simulink model "Closed_Loop_With_PID_Neural_for_Attitude_plant_predcont"  (R2018b)
settings: Solver=ode45  StartTime=0.0  StopTime=100  FixedStep=0.0001  RelTol=1e3  SampleTimeConstraint=STIndependent  EnableMultiTasking=on
undefined symbols (not defined in the file): DiscIntNeverNeededParam
libraries: dspmtrx3 x6, neural x3, vrlib x2, sharedutil x1, slrtlib x1
CloseFcn:
  | rtwprivate ssgencode ModelCloseRequest controller
settings Model: Creator=acer  LastModifiedBy=the other guy
settings SolverCC: ZeroCrossControl=DisableAll  AutoInsertRateTranBlk=on
settings DataIOCC: LimitDataPoints=on  SaveFormat=Array  SignalLoggingSaveFormat=ModelDataLogs
settings OptimizationCC: ExpressionDepthLimit=2147483647  LifeSpan=inf
settings DebuggingCC: SaveWithParameterizedLinksMsg=none  UnderspecifiedInitializationDetection=Classic  MergeDetectMultiDrivingBlocksExec=none  SolverPrmCheckMsg=warning  FcnCallInpInsideContextMsg=warning  StateNameClashWarn=warning  SFUnexpectedBacktrackingDiag=warning  SFNoUnconditionalDefaultTransitionDiag=warning  SFExecutionAtInitializationDiag=none
settings HardwareCC: ProdBitPerPointer=32  ProdBitPerSizeT=32  ProdBitPerPtrDiffT=32  ProdLargestAtomicFloat=None  ProdIntDivRoundTo=Undefined  ProdEndianess=Unspecified  ProdWordSize=32  ProdHWDeviceType=32-bit Generic
settings ModelReferenceCC: PropagateSignalLabelsOutOfModel=off
settings SFSimCC: SimUseLocalCustomCode=off
settings RTWCC: RTWUseLocalCustomCode=off
settings CodeAppCC: StateflowObjectComments=on
settings GRTTargetCC: TargetLangStandard=C89/C90 (ANSI)  GeneratePreprocessorConditionals=Disable all  CombineOutputUpdateFcns=off  GRTInterface=on
settings ConfigComp: CovMetricSettings=dw  CovHtmlReporting=on  CovSaveCumulativeToWorkspaceVar=on  CovSaveSingleToWorkspaceVar=on  CovExternalEMLEnable=off

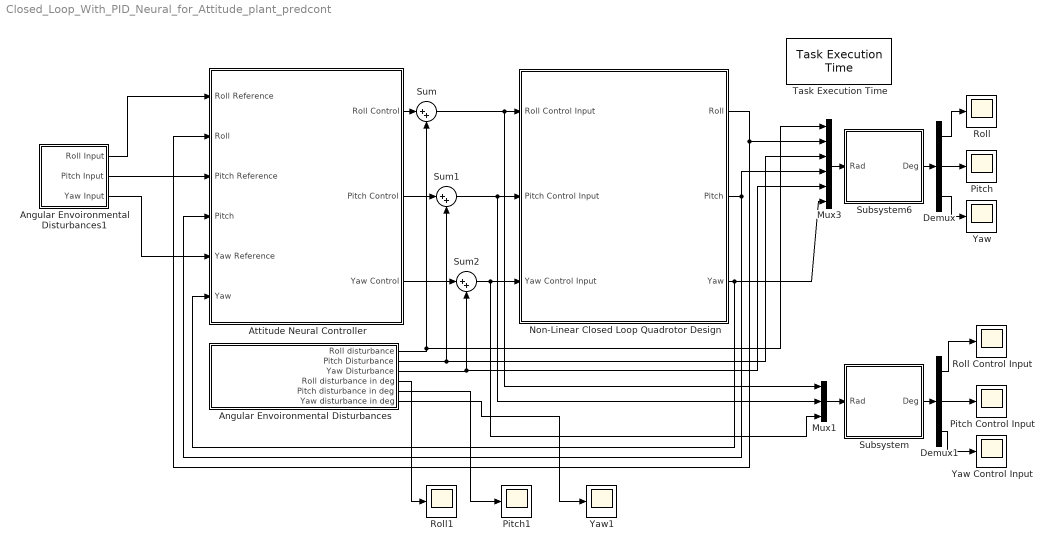
== system Closed_Loop_With_PID_Neural_for_Attitude_plant_predcont ==
  Angular Envoironmental Disturbances : Subsystem
  Angular Envoironmental Disturbances1 : Subsystem
  Attitude Neural Controller : Subsystem
  Demux : Demux  Outputs=[2,2,2]
  Demux1 : Demux  Outputs=3
  Mux1 : Mux  Inputs=3
  Mux3 : Mux  Inputs=6
  Non-Linear Closed Loop Quadrotor Design : Subsystem
  Pitch : Scope
  Pitch Control Input : Scope
  Pitch1 : Scope
  Roll : Scope
  Roll Control Input : Scope
  Roll1 : Scope
  Subsystem : Subsystem
  Subsystem6 : Subsystem
  Sum : Sum  Inputs=|++
  Sum1 : Sum  Inputs=|++
  Sum2 : Sum  Inputs=|++
  "Task Execution Time " : slrtlib/Target Management/Execution Parameters/Task Execution Time   ts=0.001
      settings: SourceProductName=Simulink Real-Time  SourceProductBaseCode=XP
  Yaw : Scope
  Yaw Control Input : Scope
  Yaw1 : Scope
  wires:
  Non-Linear Closed Loop Quadrotor Design/1(Roll) -> Mux3/2, Attitude Neural Controller/2(Roll)
  Angular Envoironmental Disturbances1/1(Roll Input) -> Attitude Neural Controller/1(Roll Reference)
  Demux1/1 -> Roll Control Input/1
  Angular Envoironmental Disturbances1/2(Pitch Input) -> Attitude Neural Controller/3(Pitch Reference)
  Non-Linear Closed Loop Quadrotor Design/2(Pitch) -> Attitude Neural Controller/4(Pitch), Mux3/4
  Demux1/2 -> Pitch Control Input/1
  Sum1/1 -> Mux1/2, Non-Linear Closed Loop Quadrotor Design/2(Pitch Control Input)
  Sum/1 -> Mux1/1, Non-Linear Closed Loop Quadrotor Design/1(Roll Control Input)
  Sum2/1 -> Mux1/3, Non-Linear Closed Loop Quadrotor Design/3(Yaw Control Input)
  Non-Linear Closed Loop Quadrotor Design/3(Yaw) -> Attitude Neural Controller/6(Yaw), Mux3/6
  Angular Envoironmental Disturbances1/3(Yaw Input) -> Attitude Neural Controller/5(Yaw Reference)
  Demux1/3 -> Yaw Control Input/1
  Mux3/1 -> Subsystem6/1(Rad)
  Subsystem6/1(Deg) -> Demux/1
  Demux/2 -> Pitch/1
  Mux1/1 -> Subsystem/1(Rad)
  Subsystem/1(Deg) -> Demux1/1
  Attitude Neural Controller/3(Yaw Control) -> Sum2/1
  Angular Envoironmental Disturbances/3(Yaw Disturbance) -> Mux3/5, Sum2/2
  Attitude Neural Controller/2(Pitch Control) -> Sum1/1
  Angular Envoironmental Disturbances/2(Pitch Disturbance) -> Mux3/3, Sum1/2
  Attitude Neural Controller/1(Roll Control) -> Sum/1
  Angular Envoironmental Disturbances/1(Roll disturbance) -> Mux3/1, Sum/2
  Demux/1 -> Roll/1
  Demux/3 -> Yaw/1
  Angular Envoironmental Disturbances/5(Pitch disturbance in deg) -> Pitch1/1
  Angular Envoironmental Disturbances/4(Roll disturbance in deg) -> Roll1/1
  Angular Envoironmental Disturbances/6(Yaw disturbance in deg) -> Yaw1/1

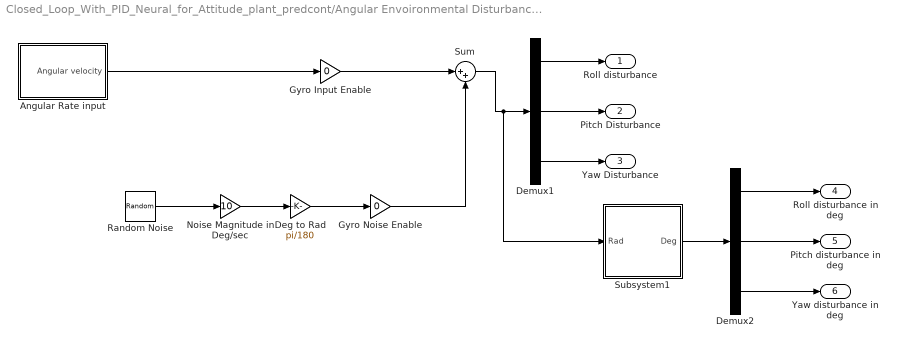
== system Closed_Loop_With_PID_Neural_for_Attitude_plant_predcont/Angular Envoironmental Disturbances ==
  Angular Rate input : Subsystem
  Deg to Rad : Gain  Gain=pi/180
  Demux1 : Demux  Outputs=3
  Demux2 : Demux  Outputs=3
  Gyro Input Enable : Gain  Gain=0
  Gyro Noise Enable : Gain  Gain=0
  Noise Magnitude in Deg/sec : Gain  Gain=10
  Random Noise : RandomNumber  Variance=0.25  SampleTime=0
  Subsystem1 : Subsystem
  Sum : Sum  Inputs=|++
  Roll disturbance : Outport
  Pitch Disturbance : Outport  Port=2
  Yaw Disturbance : Outport  Port=3
  Roll disturbance in deg : Outport  Port=4
  Pitch disturbance in deg : Outport  Port=5
  Yaw disturbance in deg : Outport  Port=6
  wires:
  Random Noise/1 -> Noise Magnitude in Deg/sec/1
  Sum/1 -> Subsystem1/1(Rad), Demux1/1
  Gyro Noise Enable/1 -> Sum/2
  Angular Rate input/1(Angular velocity) -> Gyro Input Enable/1
  Deg to Rad/1 -> Gyro Noise Enable/1
  Noise Magnitude in Deg/sec/1 -> Deg to Rad/1
  Gyro Input Enable/1 -> Sum/1
  Demux1/1 -> Roll disturbance/1
  Demux1/2 -> Pitch Disturbance/1
  Demux1/3 -> Yaw Disturbance/1
  Subsystem1/1(Deg) -> Demux2/1
  Demux2/1 -> Roll disturbance in deg/1
  Demux2/3 -> Yaw disturbance in deg/1
  Demux2/2 -> Pitch disturbance in deg/1

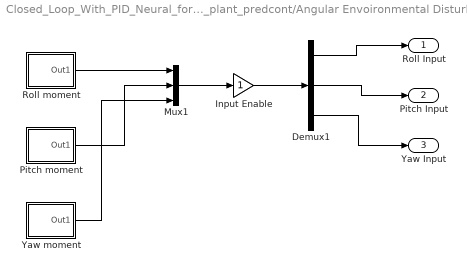
== system Closed_Loop_With_PID_Neural_for_Attitude_plant_predcont/Angular Envoironmental Disturbances1 ==
  Demux1 : Demux  Outputs=3
  Input Enable : Gain
  Mux1 : Mux  Inputs=3
  Pitch moment : Subsystem  mask(timed input){t=[0 100 100 500], u=[0 0 25 25]*pi/180}
      mask prompts: t "time values:"; u "input values"
      mask Display: plot(t,u)
  Roll moment : Subsystem  mask(timed input){t=[0 200 200 500], u=[0 0 20 20]*pi/180}
      mask prompts: t "time values:"; u "input values"
      mask Display: plot(t,u)
  Yaw moment : Subsystem  mask(timed input){t=[0 300 300 500], u=[0 0 10 10]*pi/180}
      mask prompts: t "time values:"; u "input values"
      mask Display: plot(t,u)
  Roll Input : Outport
  Pitch Input : Outport  Port=2
  Yaw Input : Outport  Port=3
  wires:
  Demux1/1 -> Roll Input/1
  Demux1/2 -> Pitch Input/1
  Demux1/3 -> Yaw Input/1
  Input Enable/1 -> Demux1/1
  Mux1/1 -> Input Enable/1
  Roll moment/1(Out1) -> Mux1/1
  Pitch moment/1(Out1) -> Mux1/2
  Yaw moment/1(Out1) -> Mux1/3

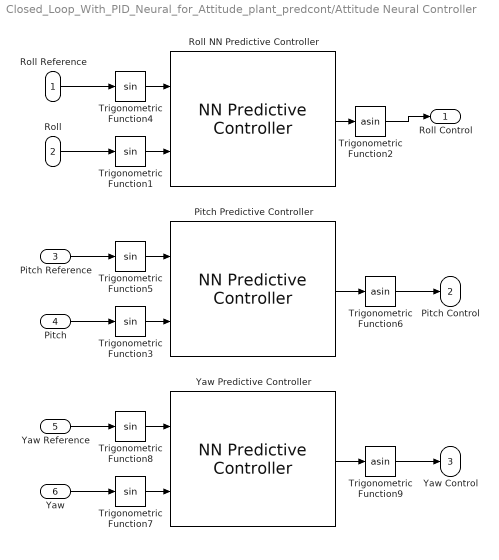
== system Closed_Loop_With_PID_Neural_for_Attitude_plant_predcont/Attitude Neural Controller ==
  Roll Reference : Inport
  Roll : Inport  Port=2
  Pitch Reference : Inport  Port=3
  Pitch : Inport  Port=4
  Yaw Reference : Inport  Port=5
  Yaw : Inport  Port=6
  Pitch Predictive Controller : neural/Control Systems/NN Predictive Controller  epochs=200  minp=-0.93969262078590832  maxp=0.93969262078590832  mint=-0.9848038138280788  maxt=0.93969262078590832  Normalize=0  IW=[0.96587729433290814 0.93651751782781034;1.3261280377593603 1.0406047962475298;0.0011576831676796625 -0.0012706400100350502;1.0232946353195504 -0.91342387371635203;-0.00083535536306784659 0.0012432394519225826]  LW1_2=[1.6026008157208218 -0.53757850024244314;0.50563527900515637 -0.47898980759277515;0.57982431361193076 -0.29736660528391951;-0.58640385446178644 1.2732333327215009;0.96805405246610521 -0.42411790933178456]  LW2_1=[-0.00084623774505455203 0.0002913868196986156 3.2621095367696893 0.027883845918589972 0.86605182305698836]  B1=[-2.0761061746421809;-1.1894731378620453;-0.39389376427834033;-2.0589212852191809;0.97157813137408788]  B2=0.59971462731666403  max_i_int=0  min_i_int=0  limit_output=0  max_output=0  min_output=0  Use_Previous_Weights=1  N2=4  Nu=4  Ts=1  rho=0.002  alpha=0.0005  csrchfun=csrchbac  maxiter=2  S1=5  Ni=2  Nj=2  sim_file=0  trainfun=trainlm  Use_validation=1  Use_Testing=1  max_i=1  min_i=-1  sam_training=0
      settings: SourceProductName=Deep Learning Toolbox  SourceProductBaseCode=NN
  Roll NN Predictive Controller : neural/Control Systems/NN Predictive Controller  epochs=200  minp=-0.93969262078590832  maxp=0.93969262078590832  mint=-0.9848038138280788  maxt=0.93969262078590832  Normalize=0  IW=[0.96587729433290814 0.93651751782781034;1.3261280377593603 1.0406047962475298;0.0011576831676796625 -0.0012706400100350502;1.0232946353195504 -0.91342387371635203;-0.00083535536306784659 0.0012432394519225826]  LW1_2=[1.6026008157208218 -0.53757850024244314;0.50563527900515637 -0.47898980759277515;0.57982431361193076 -0.29736660528391951;-0.58640385446178644 1.2732333327215009;0.96805405246610521 -0.42411790933178456]  LW2_1=[-0.00084623774505455203 0.0002913868196986156 3.2621095367696893 0.027883845918589972 0.86605182305698836]  B1=[-2.0761061746421809;-1.1894731378620453;-0.39389376427834033;-2.0589212852191809;0.97157813137408788]  B2=0.59971462731666403  max_i_int=0  min_i_int=0  limit_output=0  max_output=0  min_output=0  Use_Previous_Weights=1  N2=4  Nu=4  Ts=1  rho=0.002  alpha=0.0005  csrchfun=csrchbac  maxiter=2  S1=5  Ni=2  Nj=2  sim_file=0  trainfun=trainlm  Use_validation=1  Use_Testing=1  max_i=1  min_i=-1  sam_training=0
      settings: SourceProductName=Deep Learning Toolbox  SourceProductBaseCode=NN
  Trigonometric Function{1,3..5,7..8} (6 alike) : Trigonometry
  Trigonometric Function2 : Trigonometry  Operator=asin  OutputSignalType=real
  Trigonometric Function6 : Trigonometry  Operator=asin  OutputSignalType=real
  Trigonometric Function9 : Trigonometry  Operator=asin  OutputSignalType=real
  Yaw Predictive Controller : neural/Control Systems/NN Predictive Controller  epochs=200  minp=-0.93969262078590832  maxp=0.93969262078590832  mint=-0.9848038138280788  maxt=0.93969262078590832  Normalize=0  IW=[0.96587729433290814 0.93651751782781034;1.3261280377593603 1.0406047962475298;0.0011576831676796625 -0.0012706400100350502;1.0232946353195504 -0.91342387371635203;-0.00083535536306784659 0.0012432394519225826]  LW1_2=[1.6026008157208218 -0.53757850024244314;0.50563527900515637 -0.47898980759277515;0.57982431361193076 -0.29736660528391951;-0.58640385446178644 1.2732333327215009;0.96805405246610521 -0.42411790933178456]  LW2_1=[-0.00084623774505455203 0.0002913868196986156 3.2621095367696893 0.027883845918589972 0.86605182305698836]  B1=[-2.0761061746421809;-1.1894731378620453;-0.39389376427834033;-2.0589212852191809;0.97157813137408788]  B2=0.59971462731666403  max_i_int=0  min_i_int=0  limit_output=0  max_output=0  min_output=0  Use_Previous_Weights=1  N2=4  Nu=4  Ts=1  rho=0.002  alpha=0.0005  csrchfun=csrchbac  maxiter=2  S1=5  Ni=2  Nj=2  sim_file=0  trainfun=trainlm  Use_validation=1  Use_Testing=1  max_i=1  min_i=-1  sam_training=0
      settings: SourceProductName=Deep Learning Toolbox  SourceProductBaseCode=NN
  Roll Control : Outport
  Pitch Control : Outport  Port=2
  Yaw Control : Outport  Port=3
  wires:
  Trigonometric Function5/1 -> Pitch Predictive Controller/1
  Roll NN Predictive Controller/1 -> Trigonometric Function2/1
  Trigonometric Function1/1 -> Roll NN Predictive Controller/2
  Trigonometric Function4/1 -> Roll NN Predictive Controller/1
  Trigonometric Function3/1 -> Pitch Predictive Controller/2
  Trigonometric Function6/1 -> Pitch Control/1
  Trigonometric Function2/1 -> Roll Control/1
  Pitch Predictive Controller/1 -> Trigonometric Function6/1
  Pitch/1 -> Trigonometric Function3/1
  Pitch Reference/1 -> Trigonometric Function5/1
  Roll Reference/1 -> Trigonometric Function4/1
  Roll/1 -> Trigonometric Function1/1
  Yaw/1 -> Trigonometric Function7/1
  Yaw Reference/1 -> Trigonometric Function8/1
  Yaw Predictive Controller/1 -> Trigonometric Function9/1
  Trigonometric Function7/1 -> Yaw Predictive Controller/2
  Trigonometric Function8/1 -> Yaw Predictive Controller/1
  Trigonometric Function9/1 -> Yaw Control/1

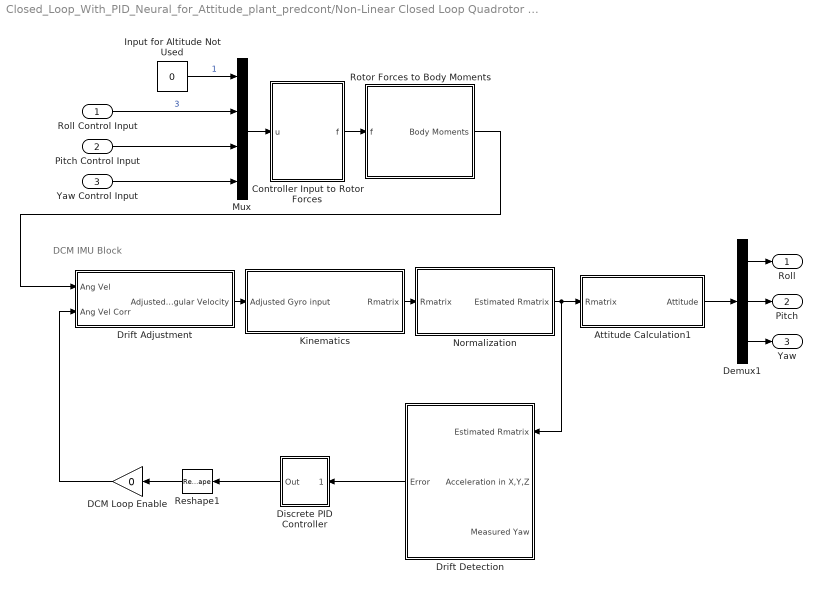
== system Closed_Loop_With_PID_Neural_for_Attitude_plant_predcont/Non-Linear Closed Loop Quadrotor Design ==
  note: DCM IMU Block
  Roll Control Input : Inport
  Pitch Control Input : Inport  Port=2
  Yaw Control Input : Inport  Port=3
  Attitude Calculation1 : Subsystem
  Controller Input to Rotor Forces : Subsystem
  DCM Loop Enable : Gain  Gain=0
  Demux1 : Demux  Outputs=3
  Discrete PID Controller : Subsystem  AncestorBlock=|  DialogController=POWERSYS.PowerSysDialog  mask(Discrete PID Controller){Kp=5, Ki=2, Kd=0, TcD=0, Par_Limits=[1e6 -1e6], Init=0, Ts=1}
      | powerlib_extras/Discrete 
      | Control Blocks/Discrete
      | PID Controller
      mask prompts: Kp "Proportional gain (Kp):"; Ki "Integral gain (Ki):"; Kd "Derivative gain (Kd):"; TcD "Time constant for derivative (s):"; Par_Limits "Output limits: [ Upper   Lower ]"; Init "Output initial value:"; Ts "Sample time:"
      mask help: This block implements a discrete PID controller.
      mask init:
      | UpperLimit=Par_Limits(1);
      | LowerLimit=Par_Limits(2);
      | power_initmask();
      mask Help: This block is part of a subset of blocks in the Extras library that does not have documentation associated with it, other than the block mask description.
      mask Display: disp('PID');
  Drift Adjustment : Subsystem
  Drift Detection : Subsystem
  Input for Altitude Not Used : Constant  Value=0
  Kinematics : Subsystem
  Mux : Mux
  Normalization : Subsystem
  Reshape1 : Reshape  OutputDimensionality=Column vector (2-D)
  Rotor Forces to Body Moments : Subsystem
  Roll : Outport
  Pitch : Outport  Port=2
  Yaw : Outport  Port=3
  wires:
  Controller Input to Rotor Forces/1(f) -> Rotor Forces to Body Moments/1(f)
  Attitude Calculation1/1(Attitude) -> Demux1/1
  Input for Altitude Not Used/1 -> Mux/1  "1"
  Roll Control Input/1 -> Mux/2  "3"
  Mux/1 -> Controller Input to Rotor Forces/1(u)
  Demux1/1 -> Roll/1
  Pitch Control Input/1 -> Mux/3
  Demux1/2 -> Pitch/1
  Yaw Control Input/1 -> Mux/4
  Demux1/3 -> Yaw/1
  Kinematics/1(Rmatrix) -> Normalization/1(Rmatrix)
  Normalization/1(Estimated Rmatrix) -> Attitude Calculation1/1(Rmatrix), Drift Detection/1(Estimated Rmatrix)
  DCM Loop Enable/1 -> Drift Adjustment/2(Ang Vel Corr)
  Reshape1/1 -> DCM Loop Enable/1
  Discrete PID Controller/1(Out) -> Reshape1/1
  Drift Detection/1(Error) -> Discrete PID Controller/1(Error)
  Rotor Forces to Body Moments/1(Body Moments) -> Drift Adjustment/1(Ang Vel)
  Drift Adjustment/1(Adjusted Angular Velocity) -> Kinematics/1(Adjusted Gyro input)

== system Closed_Loop_With_PID_Neural_for_Attitude_plant_predcont/Subsystem ==
  Rad : Inport
  Constant : Constant  Value=180/pi
  Product1 : Product  RndMeth=Zero
  Deg : Outport
  wires:
  Constant/1 -> Product1/2
  Rad/1 -> Product1/1
  Product1/1 -> Deg/1

== system Closed_Loop_With_PID_Neural_for_Attitude_plant_predcont/Subsystem6 ==
  Rad : Inport
  Constant : Constant  Value=180/pi
  Product1 : Product  RndMeth=Zero
  Deg : Outport
  wires:
  Constant/1 -> Product1/2
  Rad/1 -> Product1/1
  Product1/1 -> Deg/1

== system Closed_Loop_With_PID_Neural_for_Attitude_plant_predcont/Angular Envoironmental Disturbances/Angular Rate input ==
  Mux : Mux  Inputs=3
  Pitch moment : Subsystem  mask(timed input){t=[0 100 100 200 200 300 300 400 400 500], u=[0 0 30 30 0 0 -30 -30 0 0]*pi/180}
      mask prompts: t "time values:"; u "input values"
      mask Display: plot(t,u)
  Roll moment : Subsystem  mask(timed input){t=[0 100 100 200 200 300 300 400 400 550]-50, u=[0 0 40 40 0 0 -40 -40 0 0]*pi/180}
      mask prompts: t "time values:"; u "input values"
      mask Display: plot(t,u)
  Yaw moment : Subsystem  mask(timed input){t=[0 200 200 300 300 400 400 500 500 525]-25, u=[0 0 45 45 0 0 -45 -45 0 0]*pi/180}
      mask prompts: t "time values:"; u "input values"
      mask Display: plot(t,u)
  Angular velocity : Outport
  wires:
  Roll moment/1(Out1) -> Mux/1
  Pitch moment/1(Out1) -> Mux/2
  Yaw moment/1(Out1) -> Mux/3
  Mux/1 -> Angular velocity/1

== system Closed_Loop_With_PID_Neural_for_Attitude_plant_predcont/Angular Envoironmental Disturbances/Subsystem1 ==
  Rad : Inport
  Constant : Constant  Value=180/pi
  Product1 : Product  RndMeth=Zero
  Deg : Outport
  wires:
  Constant/1 -> Product1/2
  Rad/1 -> Product1/1
  Product1/1 -> Deg/1

== system Closed_Loop_With_PID_Neural_for_Attitude_plant_predcont/Angular Envoironmental Disturbances1/Pitch moment ==
  From Workspace : FromWorkspace  VariableName=[t',u']  SampleTime=0
  Out1 : Outport
  wires:
  From Workspace/1 -> Out1/1

== system Closed_Loop_With_PID_Neural_for_Attitude_plant_predcont/Angular Envoironmental Disturbances1/Roll moment ==
  From Workspace : FromWorkspace  VariableName=[t',u']  SampleTime=0
  Out1 : Outport
  wires:
  From Workspace/1 -> Out1/1

== system Closed_Loop_With_PID_Neural_for_Attitude_plant_predcont/Angular Envoironmental Disturbances1/Yaw moment ==
  From Workspace : FromWorkspace  VariableName=[t',u']  SampleTime=0
  Out1 : Outport
  wires:
  From Workspace/1 -> Out1/1

== system Closed_Loop_With_PID_Neural_for_Attitude_plant_predcont/Non-Linear Closed Loop Quadrotor Design/Attitude Calculation1 ==
  Rmatrix : Inport
  Embedded MATLAB Function1 : MATLAB Function  TreatAsAtomicUnit=on
  Mux : Mux  Inputs=3
  Attitude : Outport
  wires:
  Embedded MATLAB Function1/1(Roll) -> Mux/1
  Mux/1 -> Attitude/1
  Rmatrix/1 -> Embedded MATLAB Function1/1(R_mat)
  Embedded MATLAB Function1/2(Pitch) -> Mux/2
  Embedded MATLAB Function1/3(Yaw) -> Mux/3

== system Closed_Loop_With_PID_Neural_for_Attitude_plant_predcont/Non-Linear Closed Loop Quadrotor Design/Controller Input to Rotor Forces ==
  u : Inport
  Matrix Multiply : Product  Multiplication=Matrix(*)
  inv(plant_model) : Constant  Value=|  VectorParams1D=off
      | [  -0.2500         0   -0.5000   -0.2500
      |  ;  -0.2500   -0.5000         0    0.2500
      |   ; -0.2500         0    0.5000   -0.2500
      |   ; -0.2500    0.5000         0    0.2500
      | ]
  f : Outport
  wires:
  inv(plant_model)/1 -> Matrix Multiply/1
  Matrix Multiply/1 -> f/1
  u/1 -> Matrix Multiply/2

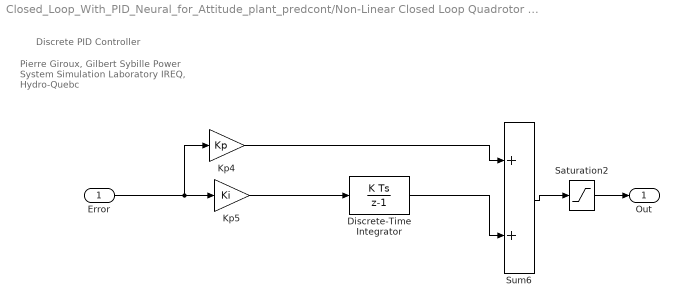
== system Closed_Loop_With_PID_Neural_for_Attitude_plant_predcont/Non-Linear Closed Loop Quadrotor Design/Discrete PID Controller ==
  note: Pierre Giroux, Gilbert Sybille
      | Power System Simulation Laboratory
      | IREQ, Hydro-Quebc
  note: Discrete PID Controller
  Error : Inport
  Discrete-Time Integrator : DiscreteIntegrator  InitialCondition=Init  SampleTime=Ts  LimitOutput=on  UpperSaturationLimit=UpperLimit  LowerSaturationLimit=LowerLimit  ICPrevOutput=DiscIntNeverNeededParam  ICPrevScaledInput=DiscIntNeverNeededParam
  Kp4 : Gain  Gain=Kp  SaturateOnIntegerOverflow=on  OutDataTypeStr=Inherit: Same as input  ParamDataTypeStr=Inherit: Same as input
  Kp5 : Gain  Gain=Ki  SaturateOnIntegerOverflow=on  OutDataTypeStr=Inherit: Same as input  ParamDataTypeStr=Inherit: Same as input
  Saturation2 : Saturate  UpperLimit=UpperLimit  LowerLimit=LowerLimit
  Sum6 : Sum  SaturateOnIntegerOverflow=on  InputSameDT=on  OutDataTypeStr=Inherit: Same as first input
  Out : Outport  InitialOutput=0
  wires:
  Error/1 -> Kp4/1, Kp5/1
  Sum6/1 -> Saturation2/1
  Kp5/1 -> Discrete-Time Integrator/1
  Kp4/1 -> Sum6/1
  Discrete-Time Integrator/1 -> Sum6/2
  Saturation2/1 -> Out/1

== system Closed_Loop_With_PID_Neural_for_Attitude_plant_predcont/Non-Linear Closed Loop Quadrotor Design/Drift Adjustment ==
  Ang Vel : Inport
  Ang Vel Corr : Inport  Port=2
  Sum : Sum  Inputs=|+-
  Adjusted Angular Velocity : Outport
  wires:
  Ang Vel/1 -> Sum/1
  Sum/1 -> Adjusted Angular Velocity/1
  Ang Vel Corr/1 -> Sum/2

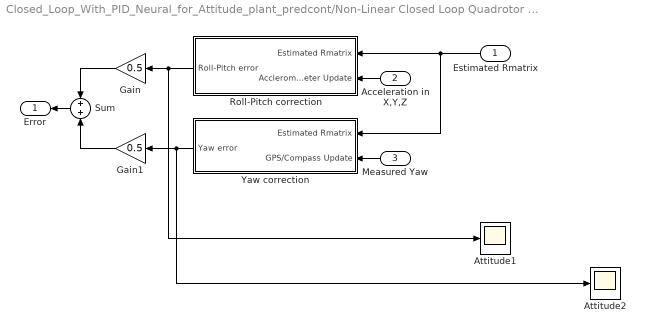
== system Closed_Loop_With_PID_Neural_for_Attitude_plant_predcont/Non-Linear Closed Loop Quadrotor Design/Drift Detection ==
  Estimated Rmatrix : Inport
  Acceleration in X,Y,Z : Inport  Port=2
  Measured Yaw : Inport  Port=3
  Attitude1 : Scope
  Attitude2 : Scope
  Gain : Gain  Gain=0.5
  Gain1 : Gain  Gain=0.5
  Roll-Pitch correction : Subsystem
  Sum : Sum
  Yaw correction : Subsystem
  Error : Outport
  wires:
  Roll-Pitch correction/1(Roll-Pitch error) -> Attitude1/1, Gain/1
  Yaw correction/1(Yaw error) -> Attitude2/1, Gain1/1
  Estimated Rmatrix/1 -> Roll-Pitch correction/1(Estimated Rmatrix), Yaw correction/1(Estimated Rmatrix)
  Acceleration in X,Y,Z/1 -> Roll-Pitch correction/2(Acclerometer Update)
  Measured Yaw/1 -> Yaw correction/2(GPS/Compass Update)
  Sum/1 -> Error/1
  Gain/1 -> Sum/1
  Gain1/1 -> Sum/2

== system Closed_Loop_With_PID_Neural_for_Attitude_plant_predcont/Non-Linear Closed Loop Quadrotor Design/Kinematics ==
  Adjusted Gyro input : Inport
  Demux : Demux  Outputs=3
  Embedded MATLAB Function : MATLAB Function  TreatAsAtomicUnit=on
  Memory : Memory
  Rmatrix : Outport
  wires:
  Demux/1 -> Embedded MATLAB Function/1(R_rate)
  Demux/2 -> Embedded MATLAB Function/2(P_rate)
  Demux/3 -> Embedded MATLAB Function/3(Y_rate)
  Embedded MATLAB Function/1(R_t) -> Memory/1, Rmatrix/1
  Memory/1 -> Embedded MATLAB Function/4(R_t_i)
  Adjusted Gyro input/1 -> Demux/1

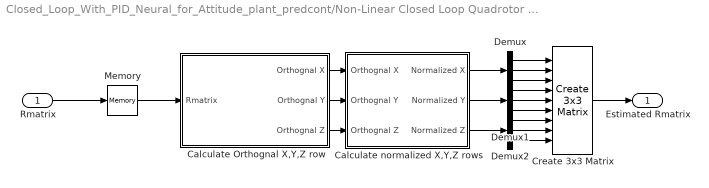
== system Closed_Loop_With_PID_Neural_for_Attitude_plant_predcont/Non-Linear Closed Loop Quadrotor Design/Normalization ==
  Rmatrix : Inport
  Calculate Orthognal X,Y,Z row : Subsystem
  Calculate normalized X,Y,Z rows : Subsystem
  Create 3x3 Matrix : sharedutil/Create 3x3 Matrix  aMode=aMode
  Demux : Demux  Outputs=3
  Demux1 : Demux  Outputs=3
  Demux2 : Demux  Outputs=3
  Memory : Memory
  Estimated Rmatrix : Outport
  wires:
  Calculate normalized X,Y,Z rows/1(Normalized X) -> Demux/1
  Calculate normalized X,Y,Z rows/2(Normalized Y) -> Demux1/1
  Calculate normalized X,Y,Z rows/3(Normalized Z) -> Demux2/1
  Demux/1 -> Create 3x3 Matrix/1
  Demux/2 -> Create 3x3 Matrix/2
  Demux/3 -> Create 3x3 Matrix/3
  Demux1/1 -> Create 3x3 Matrix/4
  Demux1/2 -> Create 3x3 Matrix/5
  Demux1/3 -> Create 3x3 Matrix/6
  Demux2/1 -> Create 3x3 Matrix/7
  Demux2/2 -> Create 3x3 Matrix/8
  Demux2/3 -> Create 3x3 Matrix/9
  Calculate Orthognal X,Y,Z row/1(Orthognal X) -> Calculate normalized X,Y,Z rows/1(Orthognal X)
  Calculate Orthognal X,Y,Z row/2(Orthognal Y) -> Calculate normalized X,Y,Z rows/2(Orthognal Y)
  Calculate Orthognal X,Y,Z row/3(Orthognal Z) -> Calculate normalized X,Y,Z rows/3(Orthognal Z)
  Rmatrix/1 -> Memory/1
  Create 3x3 Matrix/1 -> Estimated Rmatrix/1
  Memory/1 -> Calculate Orthognal X,Y,Z row/1(Rmatrix)

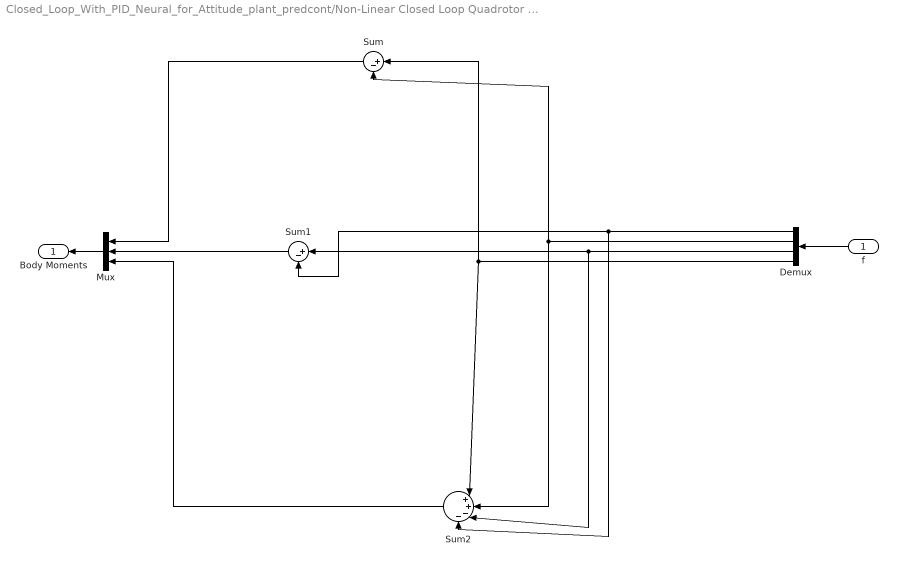
== system Closed_Loop_With_PID_Neural_for_Attitude_plant_predcont/Non-Linear Closed Loop Quadrotor Design/Rotor Forces to Body Moments ==
  f : Inport
  Demux : Demux
  Mux : Mux  Inputs=3
  Sum : Sum  Inputs=|+-
  Sum1 : Sum  Inputs=|+-
  Sum2 : Sum  Inputs=|++--
  Body Moments : Outport
  wires:
  Sum/1 -> Mux/1
  Sum1/1 -> Mux/2
  Sum2/1 -> Mux/3
  f/1 -> Demux/1
  Mux/1 -> Body Moments/1
  Demux/1 -> Sum1/2, Sum2/4
  Demux/2 -> Sum2/2, Sum/2
  Demux/3 -> Sum1/1, Sum2/3
  Demux/4 -> Sum2/1, Sum/1

== system Closed_Loop_With_PID_Neural_for_Attitude_plant_predcont/Angular Envoironmental Disturbances/Angular Rate input/Pitch moment ==
  From Workspace : FromWorkspace  VariableName=[t',u']  SampleTime=0
  Out1 : Outport
  wires:
  From Workspace/1 -> Out1/1

== system Closed_Loop_With_PID_Neural_for_Attitude_plant_predcont/Angular Envoironmental Disturbances/Angular Rate input/Roll moment ==
  From Workspace : FromWorkspace  VariableName=[t',u']  SampleTime=0
  Out1 : Outport
  wires:
  From Workspace/1 -> Out1/1

== system Closed_Loop_With_PID_Neural_for_Attitude_plant_predcont/Angular Envoironmental Disturbances/Angular Rate input/Yaw moment ==
  From Workspace : FromWorkspace  VariableName=[t',u']  SampleTime=0
  Out1 : Outport
  wires:
  From Workspace/1 -> Out1/1

== system Closed_Loop_With_PID_Neural_for_Attitude_plant_predcont/Non-Linear Closed Loop Quadrotor Design/Drift Detection/Roll-Pitch correction ==
  Estimated Rmatrix : Inport
  Acclerometer Update : Inport  Port=2
  Cross Product : vrlib/Utilities/Cross Product
      settings: SourceProductBaseCode=VR
  Row 3 selection : dspmtrx3/Submatrix  RowSpan=One row  RowStartMode=Last  RowStartIndex=1  RowEndMode=Last  RowEndIndex=1  ColSpan=All columns  ColStartMode=Last  ColStartIndex=1  ColEndMode=Last  ColEndIndex=1
  Roll-Pitch error : Outport
  wires:
  Estimated Rmatrix/1 -> Row 3 selection/1
  Cross Product/1 -> Roll-Pitch error/1
  Acclerometer Update/1 -> Cross Product/2
  Row 3 selection/1 -> Cross Product/1

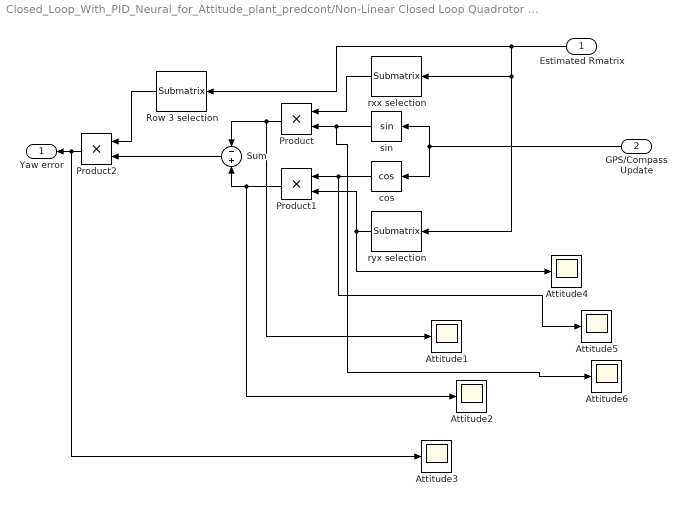
== system Closed_Loop_With_PID_Neural_for_Attitude_plant_predcont/Non-Linear Closed Loop Quadrotor Design/Drift Detection/Yaw correction ==
  Estimated Rmatrix : Inport
  GPS/Compass Update : Inport  Port=2
  Attitude{1..6} (6 alike) : Scope
  Product : Product  RndMeth=Zero
  Product1 : Product  RndMeth=Zero
  Product2 : Product  RndMeth=Zero
  Row 3 selection : dspmtrx3/Submatrix  RowSpan=One row  RowStartMode=Last  RowStartIndex=1  RowEndMode=Last  RowEndIndex=1  ColSpan=All columns  ColStartMode=First  ColStartIndex=1  ColEndMode=Last  ColEndIndex=1
  Sum : Sum  Inputs=-+
  cos : Trigonometry  Operator=cos
  rxx selection : dspmtrx3/Submatrix  RowSpan=One row  RowStartMode=First  RowStartIndex=1  RowEndMode=Last  RowEndIndex=1  ColSpan=One column  ColStartMode=First  ColStartIndex=1  ColEndMode=Last  ColEndIndex=1
  ryx selection : dspmtrx3/Submatrix  RowSpan=One row  RowStartMode=Middle  RowStartIndex=1  RowEndMode=Last  RowEndIndex=1  ColSpan=One column  ColStartMode=First  ColStartIndex=1  ColEndMode=Last  ColEndIndex=1
  sin : Trigonometry
  Yaw error : Outport
  wires:
  rxx selection/1 -> Product/1
  sin/1 -> Attitude6/1, Product/2
  ryx selection/1 -> Product1/2, Attitude4/1
  cos/1 -> Attitude5/1, Product1/1
  Product/1 -> Attitude1/1, Sum/1
  Product1/1 -> Attitude2/1, Sum/2
  Row 3 selection/1 -> Product2/1
  Sum/1 -> Product2/2
  Estimated Rmatrix/1 -> Row 3 selection/1, ryx selection/1, rxx selection/1
  GPS/Compass Update/1 -> cos/1, sin/1
  Product2/1 -> Attitude3/1, Yaw error/1

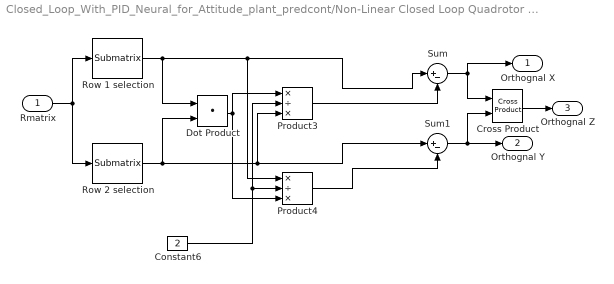
== system Closed_Loop_With_PID_Neural_for_Attitude_plant_predcont/Non-Linear Closed Loop Quadrotor Design/Normalization/Calculate Orthognal X,Y,Z row ==
  Rmatrix : Inport
  Constant6 : Constant  Value=2
  Cross Product : vrlib/Utilities/Cross Product
      settings: SourceProductBaseCode=VR
  Dot Product : DotProduct  InputSameDT=on  OutDataTypeStr=Inherit: Inherit via internal rule
  Product3 : Product  Inputs=*/*  RndMeth=Zero
  Product4 : Product  Inputs=*/*  RndMeth=Zero
  Row 1 selection : dspmtrx3/Submatrix  RowSpan=One row  RowStartMode=First  RowStartIndex=1  RowEndMode=Last  RowEndIndex=1  ColSpan=All columns  ColStartMode=First  ColStartIndex=1  ColEndMode=Last  ColEndIndex=1
  Row 2 selection : dspmtrx3/Submatrix  RowSpan=One row  RowStartMode=Middle  RowStartIndex=1  RowEndMode=Last  RowEndIndex=1  ColSpan=All columns  ColStartMode=First  ColStartIndex=1  ColEndMode=Last  ColEndIndex=1
  Sum : Sum  Inputs=|+-
  Sum1 : Sum  Inputs=|+-
  Orthognal X : Outport
  Orthognal Y : Outport  Port=2
  Orthognal Z : Outport  Port=3
  wires:
  Sum/1 -> Cross Product/1, Orthognal X/1
  Sum1/1 -> Cross Product/2, Orthognal Y/1
  Row 1 selection/1 -> Product4/1, Sum/1, Dot Product/1
  Row 2 selection/1 -> Product3/3, Sum1/1, Dot Product/2
  Constant6/1 -> Product3/2, Product4/2
  Product3/1 -> Sum/2
  Product4/1 -> Sum1/2
  Cross Product/1 -> Orthognal Z/1
  Rmatrix/1 -> Row 1 selection/1, Row 2 selection/1
  Dot Product/1 -> Product4/3, Product3/1

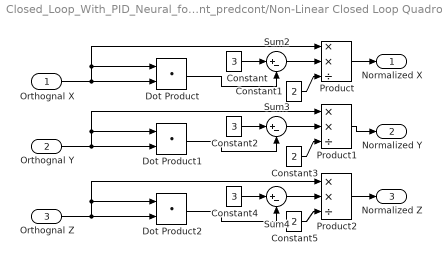
== system Closed_Loop_With_PID_Neural_for_Attitude_plant_predcont/Non-Linear Closed Loop Quadrotor Design/Normalization/Calculate normalized X,Y,Z rows ==
  Orthognal X : Inport
  Orthognal Y : Inport  Port=2
  Orthognal Z : Inport  Port=3
  Constant : Constant  Value=3
  Constant1 : Constant  Value=2
  Constant2 : Constant  Value=3
  Constant3 : Constant  Value=2
  Constant4 : Constant  Value=3
  Constant5 : Constant  Value=2
  Dot Product : DotProduct  InputSameDT=on  OutDataTypeStr=Inherit: Inherit via internal rule
  Dot Product1 : DotProduct  InputSameDT=on  OutDataTypeStr=Inherit: Inherit via internal rule
  Dot Product2 : DotProduct  InputSameDT=on  OutDataTypeStr=Inherit: Inherit via internal rule
  Product : Product  Inputs=**/  RndMeth=Zero
  Product1 : Product  Inputs=**/  RndMeth=Zero
  Product2 : Product  Inputs=**/  RndMeth=Zero
  Sum2 : Sum  Inputs=|+-
  Sum3 : Sum  Inputs=|+-
  Sum4 : Sum  Inputs=|+-
  Normalized X : Outport
  Normalized Y : Outport  Port=2
  Normalized Z : Outport  Port=3
  wires:
  Constant/1 -> Sum2/1
  Sum2/1 -> Product/2
  Constant1/1 -> Product/3
  Constant2/1 -> Sum3/1
  Sum3/1 -> Product1/2
  Constant3/1 -> Product1/3
  Constant4/1 -> Sum4/1
  Sum4/1 -> Product2/2
  Constant5/1 -> Product2/3
  Product/1 -> Normalized X/1
  Product1/1 -> Normalized Y/1
  Product2/1 -> Normalized Z/1
  Orthognal X/1 -> Dot Product/2, Dot Product/1, Product/1
  Dot Product/1 -> Sum2/2
  Orthognal Y/1 -> Dot Product1/2, Dot Product1/1, Product1/1
  Dot Product1/1 -> Sum3/2
  Orthognal Z/1 -> Dot Product2/2, Dot Product2/1, Product2/1
  Dot Product2/1 -> Sum4/2

== matlab function Closed_Loop_With_PID_Neural_for_Attitude_plant_predcont/Non-Linear Closed Loop Quadrotor Design/Kinematics/Embedded MATLAB Function ==
  data: R_rate input; R_t output; P_rate input; Y_rate input; R_t_i input
function R_t= fcn(R_rate,P_rate,Y_rate,R_t_i)
%--------------------Calculate Change in Rmatrix-------------------
dt=0.01;
a11=1;
a22=1;
a33=1;
a12=-Y_rate*dt;
a13=P_rate*dt;
a21=Y_rate*dt;
a23=-R_rate*dt;
a31=-P_rate*dt;
a32=R_rate*dt;
R_dt=[a11 a12 a13;a21 a22 a23;a31 a32 a33];
%--------------------Update Rmatrix-------------------------------
if (det(R_t_i)==0)
    R_t=[1 0 0;0 1 0;0 0 1];
else R_t=R_t_i;
end

R_t=R_t*R_dt;
% R_t=R_dt*R_t;

== matlab function Closed_Loop_With_PID_Neural_for_Attitude_plant_predcont/Non-Linear Closed Loop Quadrotor Design/Attitude Calculation1/Embedded MATLAB Function1 ==
  data: R_mat input; Roll output; Pitch output; Yaw output
function [Roll, Pitch, Yaw] = asin(R_mat)
% Roll = atan2(u(2,3),u(3,3));
% Pitch=-asin(u(1,3));
% Yaw=atan2(u(1,2),u(1,1));
Roll = atan2(R_mat(3,2),R_mat(3,3));
Pitch=-asin(R_mat(3,1));
Yaw=atan2(R_mat(2,1),R_mat(1,1));
